simulink model "Transformada_Clarke_Corrente"  (R2014a)
settings: Solver=ode45  StartTime=0.0  StopTime=0.033  MaxStep=1e-4  RelTol=1e-3
libraries: powerlib x1
settings Model: Creator=Joao  LastModifiedBy=Joao

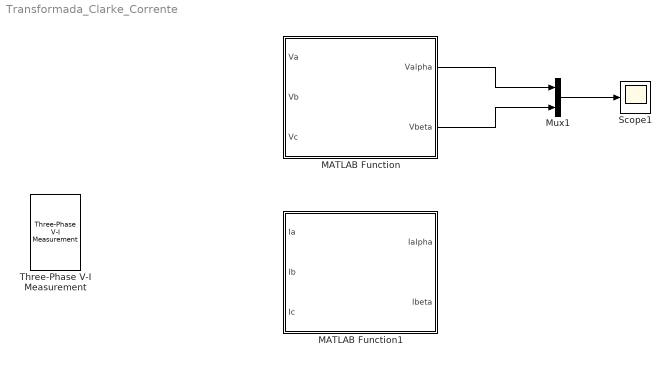
== system Transformada_Clarke_Corrente ==
  MATLAB Function : MATLAB Function  TreatAsAtomicUnit=on
  MATLAB Function1 : MATLAB Function  TreatAsAtomicUnit=on
  Mux1 : Mux  Inputs=2
  Scope1 : Scope
  Three-Phase V-I Measurement : powerlib/Measurements/Three-Phase V-I Measurement  VoltageMeasurement=phase-to-ground  SetLabelV=off  LabelV=Vabc  Vpu=off  VpuLL=off  CurrentMeasurement=yes  SetLabelI=off  LabelI=Iabc  Ipu=off  Pbase=100e6  Vbase=500e3  OutputType=Complex  PhasorSimulation=off  PSBequivalent=0
  wires:
  MATLAB Function/1(Valpha) -> Mux1/1
  MATLAB Function/2(Vbeta) -> Mux1/2
  Mux1/1 -> Scope1/1

== matlab function Transformada_Clarke_Corrente/MATLAB Function1 ==
  data: Ia input; Ialpha output; Ib input; Ic input; Ibeta output
function [Ialpha,Ibeta] = Transformada_Clarke_Corrente(Ia,Ib,Ic)
%#codegen
I = sqrt(2/3)*[1 -1/2 -1/2; 0 sqrt(3)/2 -sqrt(3)/2]*[Ia;Ib;Ic];
Ialpha = I(1,:);
Ibeta = I(2,:);

== matlab function Transformada_Clarke_Corrente/MATLAB Function ==
  data: Va input; Valpha output; Vb input; Vc input; Vbeta output
function [Valpha,Vbeta] = Transformada_Clarke_Tensao(Va,Vb,Vc)
%#codegen
V = sqrt(2/3)*[1 -1/2 -1/2; 0 sqrt(3)/2 -sqrt(3)/2]*[Va;Vb;Vc];
Valpha = V(1,:);
Vbeta = V(2,:);
